simulink library "csu_cis_camera_image_sim_lib"  (R2014b)
settings: Solver=ode45  StartTime=0.0  StopTime=10.0  RelTol=1e-3
values from neighbouring files (symbols this model uses):
  cam_intrinsic_matrix_c = [ cam_focal_length_f/cam_pixel_size  0                                  cam_image_cx ... (first row only)    [csc_cam_camera_system_prep.m]
  cam_u_matrix = [cam_u1'/norm(cam_u1) cam_u2'/norm(cam_u2) cam_u3'/norm(cam_u3) cam_u4'/norm(cam_u4)]'    [csc_cam_camera_system_prep.m]
undefined symbols (not defined in the file or in its folder): cam_extrinsic_init, cam_image_plane_norm
libraries: util_quat_lib x2, simulink x1, util_info_lib x1
settings Model: Creator=escrane  LastModifiedBy=mstewart

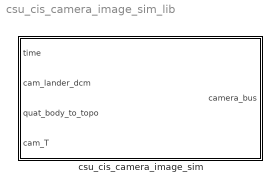
== system csu_cis_camera_image_sim_lib ==
  csu_cis_camera_image_sim : Subsystem

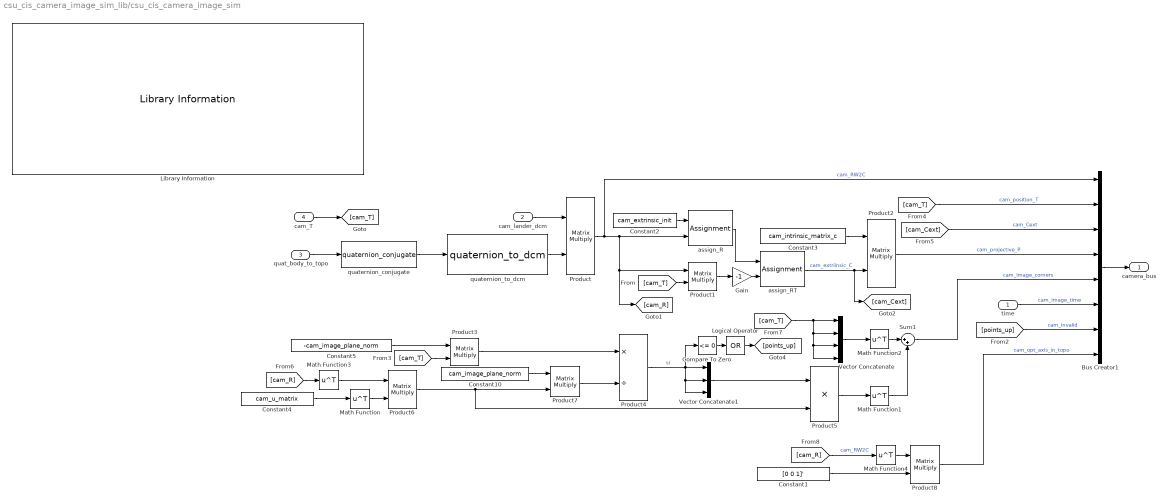
== system csu_cis_camera_image_sim_lib/csu_cis_camera_image_sim ==
  time : Inport
  cam_lander_dcm : Inport  Port=2
  quat_body_to_topo : Inport  Port=3
  cam_T : Inport  Port=4
  Bus Creator1 : BusCreator  Inputs=8
  Compare To Zero : simulink/Logic and Bit Operations/Compare To Zero  relop=<=  OutDataTypeStr=boolean
  Constant1 : Constant  Value=[0 0 1]'  VectorParams1D=off
  Constant10 : Constant  Value=cam_image_plane_norm  VectorParams1D=off
  Constant2 : Constant  Value=cam_extrinsic_init
  Constant3 : Constant  Value=cam_intrinsic_matrix_c
  Constant4 : Constant  Value=cam_u_matrix
  Constant5 : Constant  Value=-cam_image_plane_norm  VectorParams1D=off
  Gain : Gain  Gain=-1
  Library Information : util_info_lib/Library Information  owner='NONE'
  Logical Operator : Logic  Operator=OR  Inputs=1  AllPortsSameDT=off  OutDataTypeStr=boolean
  Math Function{,1..4} (5 alike) : Math  Operator=transpose  SaturateOnIntegerOverflow=on
  Product{,1..3,6..8} (7 alike) : Product  Multiplication=Matrix(*)  RndMeth=Zero
  Product4 : Product  Inputs=*/  RndMeth=Zero
  Product5 : Product  Inputs=**  RndMeth=Zero
  Sum1 : Sum  Inputs=|++
  Vector Concatenate : Concatenate  NumInputs=4  Mode=Multidimensional array  ConcatenateDimension=2
  Vector Concatenate1 : Concatenate  NumInputs=3  Mode=Multidimensional array
  assign_R : Assignment  NumberOfDimensions=2  IndexOptions=Index vector (dialog),Index vector (dialog)  Indices=[1 2 3],[1 2 3]  OutputSizes=1,1
  assign_RT : Assignment  NumberOfDimensions=2  IndexOptions=Index vector (dialog),Index vector (dialog)  Indices=[1 2 3],[4]  OutputSizes=1,1
  quaternion_conjugate : util_quat_lib/quaternion_conjugate  SystemSampleTime=-1
  quaternion_to_dcm : util_quat_lib/quaternion_to_dcm  SystemSampleTime=-1
  camera_bus : Outport
  wires:
  [points_up] -> Bus Creator1/7  "cam_invalid"
  Logical Operator/1 -> [points_up]
  Compare To Zero/1 -> Logical Operator/1
  Bus Creator1/1 -> camera_bus/1
  [cam_Cext] -> Bus Creator1/3  "cam_Cext"
  [cam_T] -> Bus Creator1/2  "cam_position_T"
  Sum1/1 -> Bus Creator1/5  "cam_image_corners"
  Product5/1 -> Math Function1/1
  Product7/1 -> Product4/2
  Product3/1 -> Product4/1
  Constant3/1 -> Product2/1
  Product2/1 -> Bus Creator1/4  "cam_projective_P"
  assign_RT/1 -> [cam_Cext], Product2/2  "cam_extriinsic_C"
  Gain/1 -> assign_RT/2
  Product1/1 -> Gain/1
  assign_R/1 -> assign_RT/1
  [cam_T] -> Product1/2
  Constant2/1 -> assign_R/1
  Product/1 -> Bus Creator1/1, assign_R/2, Product1/1, [cam_R]  "cam_RW2C"
  quat_body_to_topo/1 -> quaternion_conjugate/1
  Product6/1 -> Product5/2, Product7/2
  Constant4/1 -> Math Function/1
  [cam_R] -> Math Function3/1
  Math Function/1 -> Product6/2
  Math Function2/1 -> Sum1/1
  Vector Concatenate/1 -> Math Function2/1
  [cam_T] -> Vector Concatenate/1, Vector Concatenate/2, Vector Concatenate/3, Vector Concatenate/4
  Product4/1 -> Vector Concatenate1/1, Vector Concatenate1/2, Vector Concatenate1/3, Compare To Zero/1  "si"
  Vector Concatenate1/1 -> Product5/1
  Math Function3/1 -> Product6/1
  Constant5/1 -> Product3/1
  [cam_T] -> Product3/2
  Constant10/1 -> Product7/1
  Math Function1/1 -> Sum1/2
  quaternion_conjugate/1 -> quaternion_to_dcm/1
  time/1 -> Bus Creator1/6  "cam_image_time"
  quaternion_to_dcm/1 -> Product/2
  cam_lander_dcm/1 -> Product/1
  [cam_R] -> Math Function4/1  "cam_RW2C"
  Math Function4/1 -> Product8/1
  Constant1/1 -> Product8/2
  Product8/1 -> Bus Creator1/8  "cam_opt_axis_in_topo"
  cam_T/1 -> [cam_T]
